simulink model "waterLevel"  (R2020b)
settings: Solver=VariableStepAuto  StartTime=0.0  StopTime=10.0  RelTol=1e-3
values from neighbouring files (symbols this model uses):
  A = Kd*Kt*Rf    (= 0.1)    [main.m]
  a0 = Kt*Kp_*Rf    (= 0.25)    [main.m]
  B = Kt*Kp*Rf    (= 0.45)    [main.m]
  b0 = E    (= 0.00125)    [main.m]
  C = Ki*Kt*Rf    (= 0.75)    [main.m]
  c0 = F    (= 0.02)    [main.m]
  d0 = (J*R+b*L)*Kf + (R*b+Kt*Ke)*Kf*Rf*Ar    (= 0.08525)    [main.m]
  F = J*L*Kf+(J*R+b*L)*Kf*Rf*Ar    (= 0.02)    [main.m]
  G = (J*R+b*L)*Kf + (R*b+Kt*Ke)*Kf*Rf*Ar + Kd*Kt*Rf    (= 0.18525)    [main.m]
  H = Kf*(R*b+Kt*Ke)+Kt*Kp*Rf    (= 0.551)    [main.m]
  h0 = 1    [main.m]
  I = Ki*Kt*Rf    (= 0.75)    [main.m]
  lam = -1    [main.m]
libraries: simulink x1
settings Model: Creator=mluser  LastModifiedBy=mluser
settings DataIOCC: ReturnWorkspaceOutputs=off

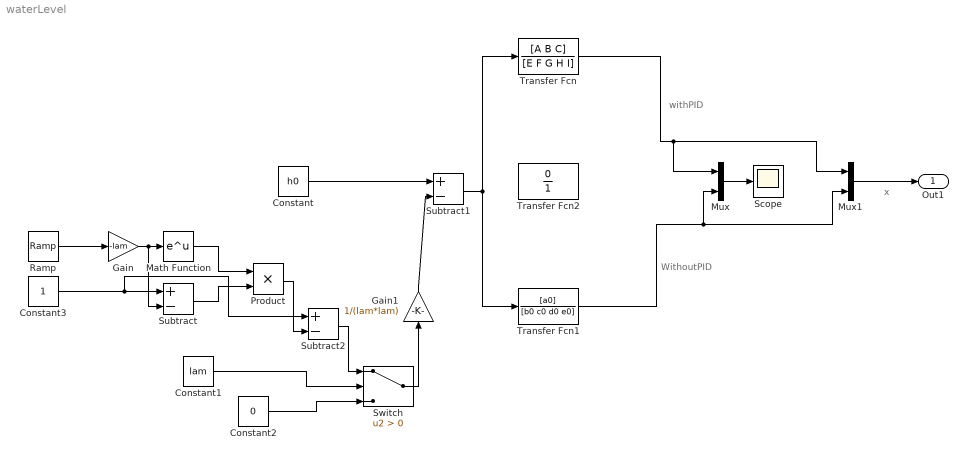
== system waterLevel ==
  note: WithoutPID
  note: x
  note: withPID
  Constant : Constant  Value=h0
  Constant1 : Constant  Value=lam
  Constant2 : Constant  Value=0
  Constant3 : Constant
  Gain : Gain  Gain=-lam
  Gain1 : Gain  Gain=1/(lam*lam)
  Math Function : Math  SaturateOnIntegerOverflow=on
  Mux : Mux  Inputs=2
  Mux1 : Mux  Inputs=2
  Product : Product
  Ramp : simulink/Sources/Ramp  slope=1  start=0  InitialOutput=0
  Scope : Scope
  Subtract : Sum  Inputs=+-
  Subtract1 : Sum  Inputs=+-
  Subtract2 : Sum  Inputs=+-
  Switch : Switch  Criteria=u2 > Threshold
  Transfer Fcn : TransferFcn  Numerator=[A B C]  Denominator=[E F G H I]
  Transfer Fcn1 : TransferFcn  Numerator=[a0]  Denominator=[b0 c0 d0 e0]
  Transfer Fcn2 : TransferFcn  Numerator=[0]  Denominator=[1]
  Out1 : Outport  SignalName=x
  wires:
  Transfer Fcn/1 -> Mux1/1, Mux/1
  Subtract1/1 -> Transfer Fcn1/1, Transfer Fcn/1
  Transfer Fcn1/1 -> Mux/2, Mux1/2
  Mux/1 -> Scope/1
  Mux1/1 -> Out1/1
  Ramp/1 -> Gain/1
  Gain/1 -> Subtract/2, Math Function/1
  Math Function/1 -> Product/1
  Constant/1 -> Subtract1/1
  Subtract2/1 -> Switch/1
  Constant1/1 -> Switch/2
  Constant2/1 -> Switch/3
  Switch/1 -> Gain1/1
  Constant3/1 -> Subtract/1, Subtract2/1
  Subtract/1 -> Product/2
  Product/1 -> Subtract2/2
  Gain1/1 -> Subtract1/2
